simulink model "Controlled_simulink_model_optimal"  (R2017b)
settings: Solver=VariableStepAuto  StartTime=0  StopTime=5  FixedStep=0.001  MaxStep=1e-3  MinStep=1e-4  RelTol=1e-5
values from neighbouring files (symbols this model uses):
  Accel_bias = 0    [Controlled_model.m]
  Ax = 0.0    (= 0)    [Controlled_model.m]
  Ay = 0.0    (= 0)    [Controlled_model.m]
  b = 1.144e-08    [Controlled_model.m]
  d = 9.94e-10    [Controlled_model.m]
  g = 9.81    [Controlled_model.m]
  Gyro_bias = 0    [Controlled_model.m]
  Ixx = 7.5*10^(-3)    (= 0.0075)    [Controlled_model.m]
  Iyy = 7.5*10^(-3)    (= 0.0075)    [Controlled_model.m]
  Izz = 1.3*10^(-2)    (= 0.013)    [Controlled_model.m]
  Jr = 6.5*10^(-7)    (= 6.5e-07)    [Controlled_model.m]
  Kd = x(3)    [Controlled_model.m]    (also in OptPID.m)
  Ki = x(2)    [Controlled_model.m]    (also in OptPID.m)
  Kp = x(1)    [Controlled_model.m]    (also in OptPID.m)
  l = 0.23    [Controlled_model.m]
  m = weight/g    (= 0.0289500509684)    [Controlled_model.m]
libraries: simulink x1
settings Model: Creator=Nicky  LastModifiedBy=Nicky
settings SolverCC: MaxConsecutiveZCs=500  ZeroCrossAlgorithm=Adaptive  AlgebraicLoopSolver=LineSearch  AutoInsertRateTranBlk=on
settings DebuggingCC: MaxConsecutiveZCsMsg=none
settings CodeAppCC: StateflowObjectComments=on
settings SimscapeCC: SimscapeNormalizeSystem=off

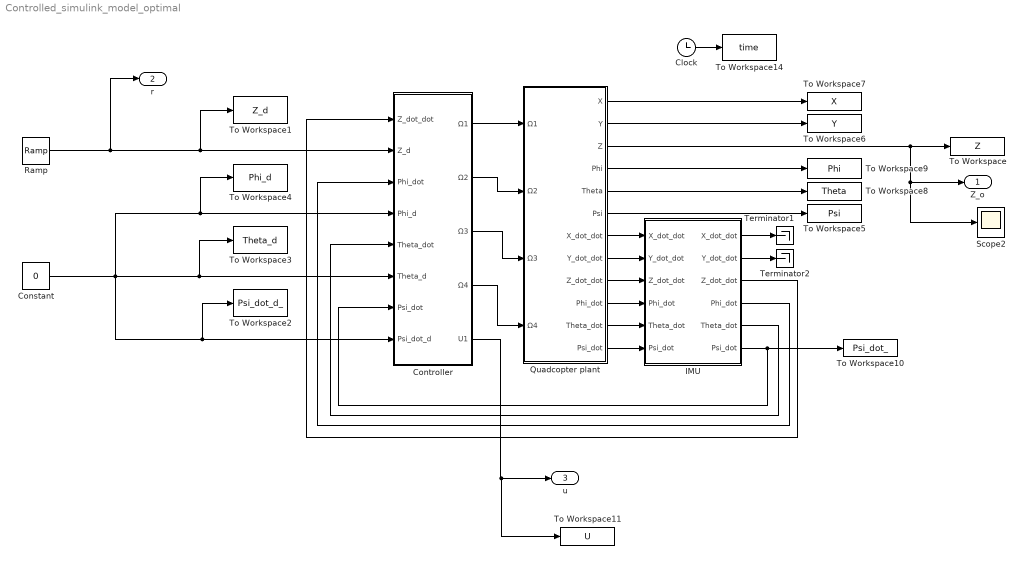
== system Controlled_simulink_model_optimal ==
  Clock : Clock
  Constant : Constant  Value=0
  Controller : Subsystem
  IMU : Subsystem
  Quadcopter plant : Subsystem
  Ramp : simulink/Sources/Ramp  slope=0  start=0  X0=-1
  Scope2 : Scope
  Terminator1 : Terminator
  Terminator2 : Terminator
  To Workspace : ToWorkspace  VariableName=Z  SampleTime=0.001
      settings: Save2DSignal=2-D array (concatenate along first dimension)
  To Workspace1 : ToWorkspace  VariableName=Z_d  SampleTime=0.001
      settings: Save2DSignal=2-D array (concatenate along first dimension)
  To Workspace10 : ToWorkspace  VariableName=Psi_dot_  SampleTime=0.001
      settings: Save2DSignal=2-D array (concatenate along first dimension)
  To Workspace11 : ToWorkspace  VariableName=U  SampleTime=0.001
      settings: Save2DSignal=2-D array (concatenate along first dimension)
  To Workspace14 : ToWorkspace  VariableName=time  SampleTime=0.001
      settings: Save2DSignal=2-D array (concatenate along first dimension)
  To Workspace2 : ToWorkspace  VariableName=Psi_dot_d_  SampleTime=0.001
      settings: Save2DSignal=2-D array (concatenate along first dimension)
  To Workspace3 : ToWorkspace  VariableName=Theta_d  SampleTime=0.001
      settings: Save2DSignal=2-D array (concatenate along first dimension)
  To Workspace4 : ToWorkspace  VariableName=Phi_d  SampleTime=0.001
      settings: Save2DSignal=2-D array (concatenate along first dimension)
  To Workspace5 : ToWorkspace  VariableName=Psi  SampleTime=0.001
      settings: Save2DSignal=2-D array (concatenate along first dimension)
  To Workspace6 : ToWorkspace  VariableName=Y  SampleTime=0.001
      settings: Save2DSignal=2-D array (concatenate along first dimension)
  To Workspace7 : ToWorkspace  VariableName=X  SampleTime=0.001
      settings: Save2DSignal=2-D array (concatenate along first dimension)
  To Workspace8 : ToWorkspace  VariableName=Theta  SampleTime=0.001
      settings: Save2DSignal=2-D array (concatenate along first dimension)
  To Workspace9 : ToWorkspace  VariableName=Phi  SampleTime=0.001
      settings: Save2DSignal=2-D array (concatenate along first dimension)
  Z_o : Outport
  r : Outport  Port=2
  "u " : Outport  Port=3
  wires:
  Clock/1 -> To Workspace14/1
  Controller/1(Ω1) -> Quadcopter plant/1(Ω1)
  Controller/2(Ω2) -> Quadcopter plant/2(Ω2)
  Controller/3(Ω3) -> Quadcopter plant/3(Ω3)
  Controller/4(Ω4) -> Quadcopter plant/4(Ω4)
  IMU/6("Psi_dot ") -> Controller/7(Psi_dot), To Workspace10/1
  IMU/5("Theta_dot ") -> Controller/5(Theta_dot)
  IMU/3("Z_dot_dot ") -> Controller/1(Z_dot_dot)
  Quadcopter plant/1(X) -> To Workspace7/1
  Quadcopter plant/2(Y) -> To Workspace6/1
  Quadcopter plant/7(X_dot_dot) -> IMU/1(X_dot_dot)
  Quadcopter plant/8("Y_dot_dot ") -> IMU/2(Y_dot_dot)
  Quadcopter plant/9(Z_dot_dot) -> IMU/3(Z_dot_dot)
  Quadcopter plant/11(Theta_dot) -> IMU/5(Theta_dot)
  Quadcopter plant/10(Phi_dot) -> IMU/4(Phi_dot)
  Quadcopter plant/12(Psi_dot) -> IMU/6(Psi_dot)
  Quadcopter plant/5(Theta) -> To Workspace8/1
  Quadcopter plant/6(Psi) -> To Workspace5/1
  IMU/1("X_dot_dot ") -> Terminator1/1
  IMU/2("Y_dot_dot ") -> Terminator2/1
  Constant/1 -> To Workspace4/1, Controller/4(Phi_d), To Workspace2/1, Controller/8(Psi_dot_d), To Workspace3/1, Controller/6(Theta_d)
  IMU/4("Phi_dot ") -> Controller/3(Phi_dot)
  Quadcopter plant/4(Phi) -> To Workspace9/1
  Ramp/1 -> r/1, To Workspace1/1, Controller/2(Z_d)
  Controller/5(U1) -> To Workspace11/1, "u "/1
  Quadcopter plant/3(Z) -> Z_o/1, Scope2/1, To Workspace/1

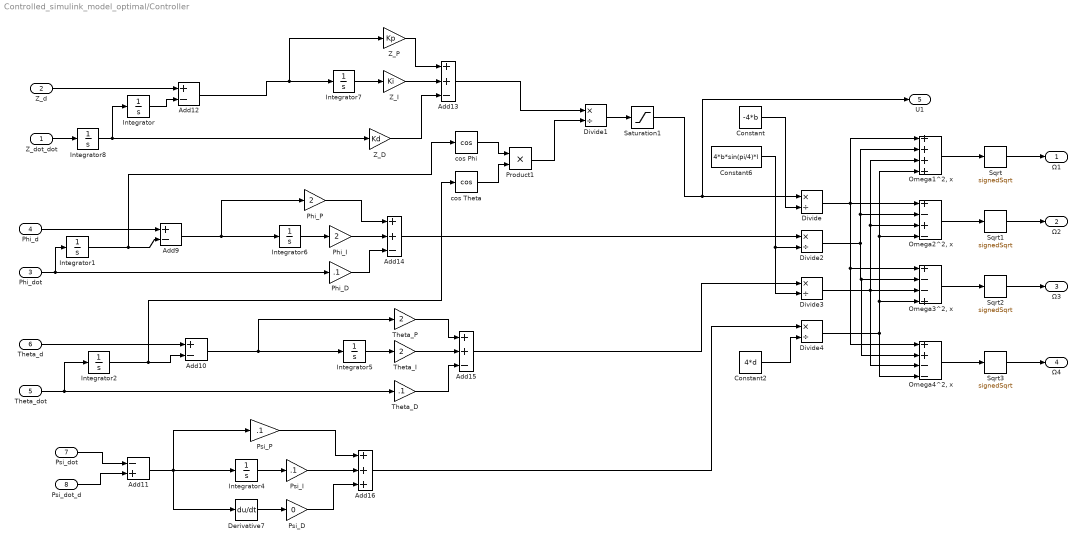
== system Controlled_simulink_model_optimal/Controller ==
  Z_dot_dot : Inport
  Z_d : Inport  Port=2
  Phi_dot : Inport  Port=3
  Phi_d : Inport  Port=4
  Theta_dot : Inport  Port=5
  Theta_d : Inport  Port=6
  Psi_dot : Inport  Port=7
  Psi_dot_d : Inport  Port=8
  Add10 : Sum  Inputs=+-
  Add11 : Sum  Inputs=-+
  Add12 : Sum  Inputs=+-
  Add13 : Sum  Inputs=++-
  Add14 : Sum  Inputs=++-
  Add15 : Sum  Inputs=++-
  Add16 : Sum  Inputs=+++
  Add9 : Sum  Inputs=+-
  Constant : Constant  Value=-4*b
  Constant2 : Constant  Value=4*d
  Constant6 : Constant  Value=4*b*sin(pi/4)*l
  Derivative7 : Derivative
  Divide{,1..4} (5 alike) : Product  Inputs=*/
  Integrator : Integrator  LimitOutput=on  UpperSaturationLimit=0
  Integrator1 : Integrator  WrapState=on
  Integrator2 : Integrator  WrapState=on
  Integrator{4..8} (5 alike) : Integrator
  "Omega1^2, x" : Sum  Inputs=++++
  "Omega2^2, x" : Sum  Inputs=+-+-
  "Omega3^2, x" : Sum  Inputs=+--+
  "Omega4^2, x" : Sum  Inputs=++--
  Phi_D : Gain  Gain=.1
  Phi_I : Gain  Gain=2
  Phi_P : Gain  Gain=2
  Product1 : Product  RndMeth=Zero
  Psi_D : Gain  Gain=0
  Psi_I : Gain  Gain=.1
  Psi_P : Gain  Gain=.1
  Saturation1 : Saturate  UpperLimit=0  LowerLimit=-inf
  Sqrt{,1..3} (4 alike) : Sqrt  Operator=signedSqrt  SaturateOnIntegerOverflow=on
  Theta_D : Gain  Gain=.1
  Theta_I : Gain  Gain=2
  Theta_P : Gain  Gain=2
  Z_D : Gain  Gain=Kd
  "Z_I " : Gain  Gain=Ki
  Z_P : Gain  Gain=Kp
  cos Phi : Trigonometry  Operator=cos
  cos Theta : Trigonometry  Operator=cos
  Ω1 : Outport
  Ω2 : Outport  Port=2
  Ω3 : Outport  Port=3
  Ω4 : Outport  Port=4
  U1 : Outport  Port=5
  wires:
  Z_D/1 -> Add13/3
  Theta_I/1 -> Add15/2
  Add12/1 -> Z_P/1, Integrator7/1
  Z_dot_dot/1 -> Integrator8/1
  Add11/1 -> Derivative7/1, Integrator4/1, Psi_P/1
  "Z_I "/1 -> Add13/2
  Theta_P/1 -> Add15/1
  Integrator4/1 -> Psi_I/1
  Integrator7/1 -> "Z_I "/1
  Add9/1 -> Integrator6/1, Phi_P/1
  Derivative7/1 -> Psi_D/1
  Psi_D/1 -> Add16/3
  Psi_I/1 -> Add16/2
  Integrator6/1 -> Phi_I/1
  cos Theta/1 -> Product1/2
  Add13/1 -> Divide1/1
  Phi_dot/1 -> Phi_D/1, Integrator1/1
  Phi_D/1 -> Add14/3
  cos Phi/1 -> Product1/1
  Divide1/1 -> Saturation1/1
  Theta_D/1 -> Add15/3
  Integrator5/1 -> Theta_I/1
  Add10/1 -> Theta_P/1, Integrator5/1
  Product1/1 -> Divide1/2
  Phi_I/1 -> Add14/2
  Theta_dot/1 -> Integrator2/1, Theta_D/1
  Phi_P/1 -> Add14/1
  Psi_P/1 -> Add16/1
  Z_P/1 -> Add13/1
  Constant6/1 -> Divide3/2, Divide2/2
  Add14/1 -> Divide2/1
  Add15/1 -> Divide3/1
  Saturation1/1 -> U1/1, Divide/1
  Constant/1 -> Divide/2
  Constant2/1 -> Divide4/2
  Add16/1 -> Divide4/1
  Sqrt/1 -> Ω1/1
  Sqrt1/1 -> Ω2/1
  Sqrt2/1 -> Ω3/1
  Sqrt3/1 -> Ω4/1
  Divide4/1 -> "Omega3^2, x"/4, "Omega2^2, x"/4, "Omega1^2, x"/4, "Omega4^2, x"/4
  Divide2/1 -> "Omega4^2, x"/2, "Omega3^2, x"/2, "Omega2^2, x"/2, "Omega1^2, x"/2
  Divide3/1 -> "Omega4^2, x"/3, "Omega3^2, x"/3, "Omega2^2, x"/3, "Omega1^2, x"/3
  Divide/1 -> "Omega4^2, x"/1, "Omega3^2, x"/1, "Omega2^2, x"/1, "Omega1^2, x"/1
  "Omega1^2, x"/1 -> Sqrt/1
  "Omega2^2, x"/1 -> Sqrt1/1
  "Omega3^2, x"/1 -> Sqrt2/1
  "Omega4^2, x"/1 -> Sqrt3/1
  Z_d/1 -> Add12/1
  Phi_d/1 -> Add9/1
  Integrator1/1 -> cos Phi/1, Add9/2
  Integrator2/1 -> cos Theta/1, Add10/2
  Theta_d/1 -> Add10/1
  Psi_dot/1 -> Add11/1
  Psi_dot_d/1 -> Add11/2
  Integrator/1 -> Add12/2
  Integrator8/1 -> Z_D/1, Integrator/1

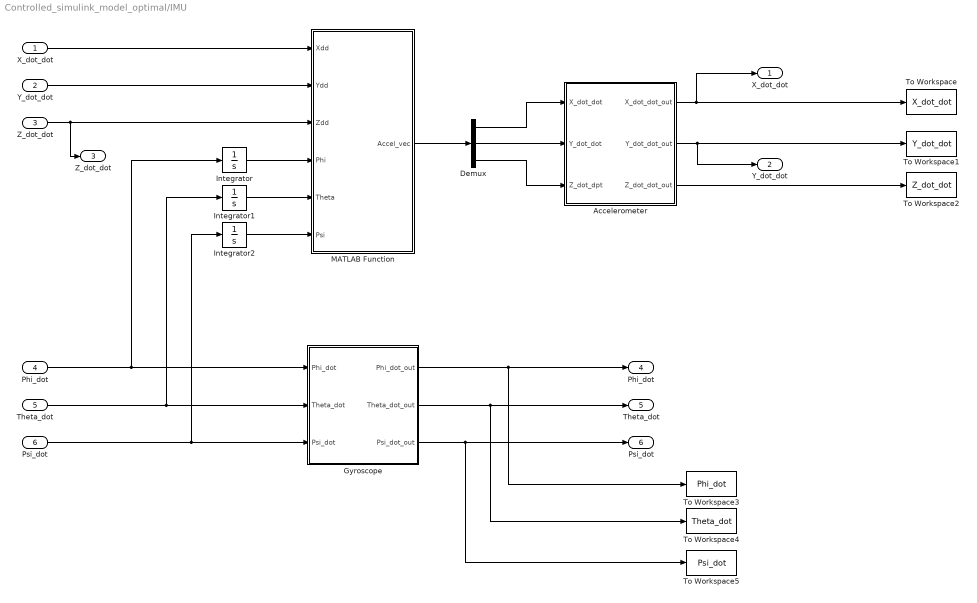
== system Controlled_simulink_model_optimal/IMU ==
  X_dot_dot : Inport
  Y_dot_dot : Inport  Port=2
  Z_dot_dot : Inport  Port=3
  Phi_dot : Inport  Port=4
  Theta_dot : Inport  Port=5
  Psi_dot : Inport  Port=6
  Accelerometer : Subsystem
  Demux : Demux  Outputs=3
  Gyroscope : Subsystem
  Integrator : Integrator  WrapState=on
  Integrator1 : Integrator  WrapState=on
  Integrator2 : Integrator
  MATLAB Function : MATLAB Function  TreatAsAtomicUnit=on
  To Workspace : ToWorkspace  VariableName=X_dot_dot  SampleTime=0.001
      settings: Save2DSignal=2-D array (concatenate along first dimension)
  To Workspace1 : ToWorkspace  VariableName=Y_dot_dot  SampleTime=0.001
      settings: Save2DSignal=2-D array (concatenate along first dimension)
  To Workspace2 : ToWorkspace  VariableName=Z_dot_dot  SampleTime=0.001
      settings: Save2DSignal=2-D array (concatenate along first dimension)
  To Workspace3 : ToWorkspace  VariableName=Phi_dot  SampleTime=0.001
      settings: Save2DSignal=2-D array (concatenate along first dimension)
  To Workspace4 : ToWorkspace  VariableName=Theta_dot  SampleTime=0.001
      settings: Save2DSignal=2-D array (concatenate along first dimension)
  To Workspace5 : ToWorkspace  VariableName=Psi_dot  SampleTime=0.001
      settings: Save2DSignal=2-D array (concatenate along first dimension)
  "X_dot_dot " : Outport
  "Y_dot_dot " : Outport  Port=2
  "Z_dot_dot " : Outport  Port=3
  "Phi_dot " : Outport  Port=4
  "Theta_dot " : Outport  Port=5
  "Psi_dot " : Outport  Port=6
  wires:
  Phi_dot/1 -> Integrator/1, Gyroscope/1(Phi_dot)
  Theta_dot/1 -> Integrator1/1, Gyroscope/2(Theta_dot)
  Psi_dot/1 -> Integrator2/1, Gyroscope/3(Psi_dot)
  Gyroscope/2(Theta_dot_out) -> "Theta_dot "/1, To Workspace4/1
  Gyroscope/1(Phi_dot_out) -> "Phi_dot "/1, To Workspace3/1
  Accelerometer/1(X_dot_dot_out) -> To Workspace/1, "X_dot_dot "/1
  Accelerometer/2(Y_dot_dot_out) -> To Workspace1/1, "Y_dot_dot "/1
  Accelerometer/3(Z_dot_dot_out) -> To Workspace2/1
  Gyroscope/3(Psi_dot_out) -> "Psi_dot "/1, To Workspace5/1
  X_dot_dot/1 -> MATLAB Function/1(Xdd)
  Y_dot_dot/1 -> MATLAB Function/2(Ydd)
  Z_dot_dot/1 -> "Z_dot_dot "/1, MATLAB Function/3(Zdd)
  Integrator/1 -> MATLAB Function/4(Phi)
  Integrator2/1 -> MATLAB Function/6(Psi)
  Integrator1/1 -> MATLAB Function/5(Theta)
  MATLAB Function/1(Accel_vec) -> Demux/1
  Demux/2 -> Accelerometer/2("Y_dot_dot ")
  Demux/1 -> Accelerometer/1(X_dot_dot)
  Demux/3 -> Accelerometer/3("Z_dot_dpt ")

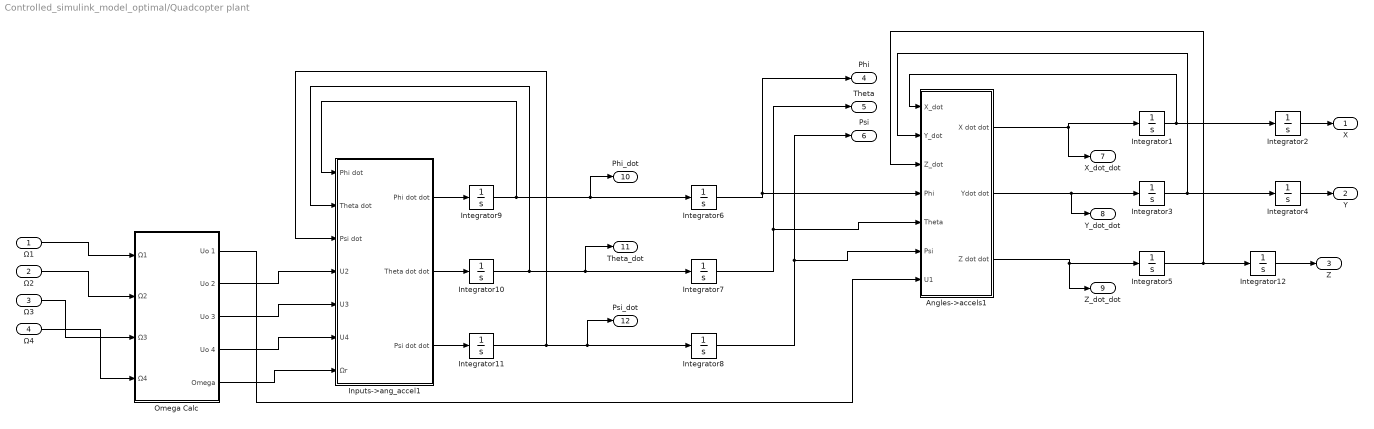
== system Controlled_simulink_model_optimal/Quadcopter plant ==
  Ω1 : Inport
  Ω2 : Inport  Port=2
  Ω3 : Inport  Port=3
  Ω4 : Inport  Port=4
  Angles->accels1 : Subsystem
  Inputs->ang_accel1 : Subsystem
  Integrator{1..5,8..9} (7 alike) : Integrator
  Integrator10 : Integrator  IgnoreLimit=on
  Integrator11 : Integrator  UpperSaturationLimit=10000  LowerSaturationLimit=-10000
  Integrator12 : Integrator  LimitOutput=on  UpperSaturationLimit=0
  Integrator6 : Integrator  WrapState=on
  Integrator7 : Integrator  WrapState=on
  Omega Calc : Subsystem
  X : Outport
  Y : Outport  Port=2
  Z : Outport  Port=3
  Phi : Outport  Port=4
  Theta : Outport  Port=5
  Psi : Outport  Port=6
  X_dot_dot : Outport  Port=7
  "Y_dot_dot " : Outport  Port=8
  Z_dot_dot : Outport  Port=9
  Phi_dot : Outport  Port=10
  Theta_dot : Outport  Port=11
  Psi_dot : Outport  Port=12
  wires:
  Integrator7/1 -> Angles->accels1/5(Theta), Theta/1
  Integrator6/1 -> Angles->accels1/4(Phi), Phi/1
  Inputs->ang_accel1/2(Theta dot dot) -> Integrator10/1
  Inputs->ang_accel1/1(Phi dot dot) -> Integrator9/1
  Inputs->ang_accel1/3(Psi dot dot) -> Integrator11/1
  Omega Calc/5(Omega) -> Inputs->ang_accel1/7(Ωr)
  Omega Calc/4(Uo 4) -> Inputs->ang_accel1/6(U4)
  Omega Calc/3(Uo 3) -> Inputs->ang_accel1/5(U3)
  Omega Calc/2(Uo 2) -> Inputs->ang_accel1/4(U2)
  Omega Calc/1(Uo 1) -> Angles->accels1/7(U1)
  Ω1/1 -> Omega Calc/1(Ω1)
  Ω2/1 -> Omega Calc/2(Ω2)
  Ω3/1 -> Omega Calc/3(Ω3)
  Ω4/1 -> Omega Calc/4(Ω4)
  Integrator9/1 -> Inputs->ang_accel1/1(Phi dot), Phi_dot/1, Integrator6/1
  Integrator11/1 -> Inputs->ang_accel1/3(Psi dot), Integrator8/1, Psi_dot/1
  Integrator10/1 -> Inputs->ang_accel1/2(Theta dot), Integrator7/1, Theta_dot/1
  Angles->accels1/1(X dot dot) -> X_dot_dot/1, Integrator1/1
  Integrator1/1 -> Angles->accels1/1(X_dot), Integrator2/1
  Integrator2/1 -> X/1
  Integrator3/1 -> Angles->accels1/2(Y_dot), Integrator4/1
  Angles->accels1/2(Ydot dot) -> "Y_dot_dot "/1, Integrator3/1
  Integrator4/1 -> Y/1
  Integrator5/1 -> Angles->accels1/3(Z_dot), Integrator12/1
  Angles->accels1/3(Z dot dot) -> Integrator5/1, Z_dot_dot/1
  Integrator12/1 -> Z/1
  Integrator8/1 -> Angles->accels1/6(Psi), Psi/1

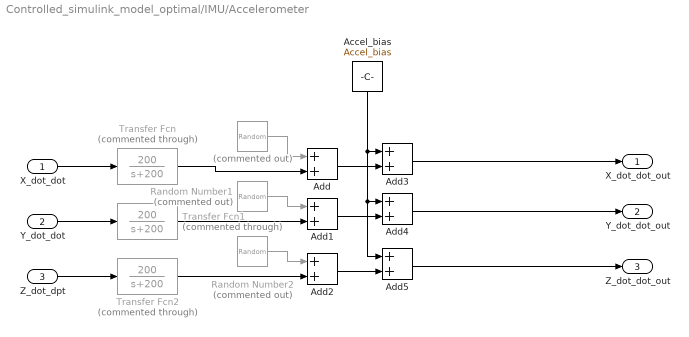
== system Controlled_simulink_model_optimal/IMU/Accelerometer ==
  X_dot_dot : Inport
  "Y_dot_dot " : Inport  Port=2
  "Z_dot_dpt " : Inport  Port=3
  " " : RandomNumber  Commented=on  Variance=0.0001  Seed=1  SampleTime=0.001
  Accel_bias : Constant  Value=Accel_bias
  Add{,1..5} (6 alike) : Sum
  Random Number1 : RandomNumber  Commented=on  Variance=0.0001  Seed=2  SampleTime=0.001
  Random Number2 : RandomNumber  Commented=on  Mean=0.000  Variance=0.0001  Seed=3  SampleTime=0.001
  Transfer Fcn : TransferFcn  Commented=through  Numerator=[200]  Denominator=[1 200]
  Transfer Fcn1 : TransferFcn  Commented=through  Numerator=[200]  Denominator=[1 200]
  Transfer Fcn2 : TransferFcn  Commented=through  Numerator=[200]  Denominator=[1 200]
  X_dot_dot_out : Outport
  Y_dot_dot_out : Outport  Port=2
  Z_dot_dot_out : Outport  Port=3
  wires:
  X_dot_dot/1 -> Transfer Fcn/1
  "Y_dot_dot "/1 -> Transfer Fcn1/1
  Accel_bias/1 -> Add5/1, Add4/1, Add3/1
  Add/1 -> Add3/2
  Add2/1 -> Add5/2
  Add1/1 -> Add4/2
  " "/1 -> Add/1
  Random Number1/1 -> Add1/1
  Random Number2/1 -> Add2/1
  "Z_dot_dpt "/1 -> Transfer Fcn2/1
  Add3/1 -> X_dot_dot_out/1
  Add4/1 -> Y_dot_dot_out/1
  Add5/1 -> Z_dot_dot_out/1
  Transfer Fcn/1 -> Add/2
  Transfer Fcn1/1 -> Add1/2
  Transfer Fcn2/1 -> Add2/2

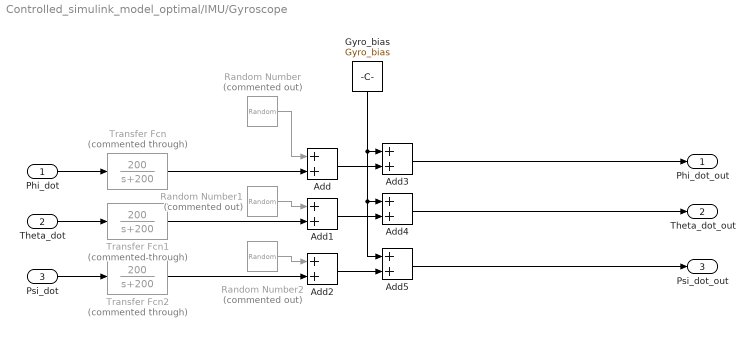
== system Controlled_simulink_model_optimal/IMU/Gyroscope ==
  Phi_dot : Inport
  Theta_dot : Inport  Port=2
  Psi_dot : Inport  Port=3
  Add{,1..5} (6 alike) : Sum
  Gyro_bias : Constant  Value=Gyro_bias
  Random Number : RandomNumber  Commented=on  Variance=0.0001  Seed=4  SampleTime=0.001
  Random Number1 : RandomNumber  Commented=on  Variance=0.0001  Seed=5  SampleTime=0.001
  Random Number2 : RandomNumber  Commented=on  Variance=0.0001  Seed=6  SampleTime=0.001
  Transfer Fcn : TransferFcn  Commented=through  Numerator=[200]  Denominator=[1 200]
  Transfer Fcn1 : TransferFcn  Commented=through  Numerator=[200]  Denominator=[1 200]
  Transfer Fcn2 : TransferFcn  Commented=through  Numerator=[200]  Denominator=[1 200]
  Phi_dot_out : Outport
  Theta_dot_out : Outport  Port=2
  Psi_dot_out : Outport  Port=3
  wires:
  Phi_dot/1 -> Transfer Fcn/1
  Theta_dot/1 -> Transfer Fcn1/1
  Psi_dot/1 -> Transfer Fcn2/1
  Add/1 -> Add3/2
  Add1/1 -> Add4/2
  Add2/1 -> Add5/2
  Gyro_bias/1 -> Add5/1, Add4/1, Add3/1
  Random Number/1 -> Add/1
  Random Number1/1 -> Add1/1
  Random Number2/1 -> Add2/1
  Add3/1 -> Phi_dot_out/1
  Add4/1 -> Theta_dot_out/1
  Add5/1 -> Psi_dot_out/1
  Transfer Fcn2/1 -> Add2/2
  Transfer Fcn1/1 -> Add1/2
  Transfer Fcn/1 -> Add/2

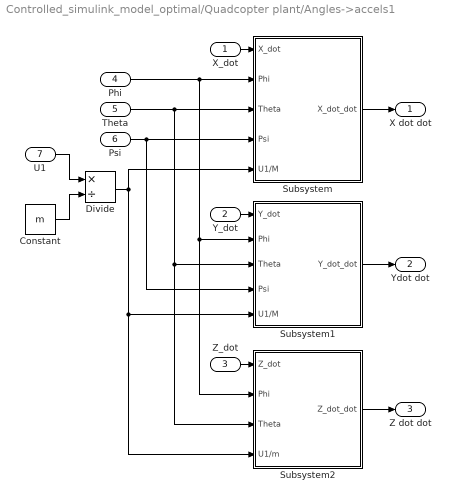
== system Controlled_simulink_model_optimal/Quadcopter plant/Angles->accels1 ==
  X_dot : Inport
  Y_dot : Inport  Port=2
  Z_dot : Inport  Port=3
  Phi : Inport  Port=4
  Theta : Inport  Port=5
  Psi : Inport  Port=6
  U1 : Inport  Port=7
  Constant : Constant  Value=m
  Divide : Product  Inputs=*/
  Subsystem : Subsystem
  Subsystem1 : Subsystem
  Subsystem2 : Subsystem
  X dot dot : Outport
  Ydot dot : Outport  Port=2
  Z dot dot : Outport  Port=3
  wires:
  Phi/1 -> Subsystem2/2(Phi), Subsystem1/2(Phi), Subsystem/2(Phi)
  U1/1 -> Divide/1
  Constant/1 -> Divide/2
  Divide/1 -> Subsystem/5(U1/M), Subsystem2/4(U1/m), Subsystem1/5(U1/M)
  Subsystem/1(X_dot_dot) -> X dot dot/1
  Subsystem1/1(Y_dot_dot) -> Ydot dot/1
  Subsystem2/1(Z_dot_dot) -> Z dot dot/1
  Theta/1 -> Subsystem2/3(Theta), Subsystem1/3(Theta), Subsystem/3(Theta)
  Psi/1 -> Subsystem1/4(Psi), Subsystem/4(Psi)
  X_dot/1 -> Subsystem/1(X_dot)
  Y_dot/1 -> Subsystem1/1(Y_dot)
  Z_dot/1 -> Subsystem2/1(Z_dot)

== system Controlled_simulink_model_optimal/Quadcopter plant/Inputs->ang_accel1 ==
  Phi dot : Inport
  Theta dot : Inport  Port=2
  Psi dot : Inport  Port=3
  U2 : Inport  Port=4
  U3 : Inport  Port=5
  U4 : Inport  Port=6
  Ωr : Inport  Port=7
  Subsystem : Subsystem
  Subsystem1 : Subsystem
  Subsystem2 : Subsystem
  Phi dot dot : Outport
  Theta dot dot : Outport  Port=2
  Psi dot dot : Outport  Port=3
  wires:
  U3/1 -> Subsystem2/3(U3)
  U4/1 -> Subsystem1/3(U4)
  Subsystem/1(Phi_dot_dot) -> Phi dot dot/1
  U2/1 -> Subsystem/1(U2)
  Ωr/1 -> Subsystem/4(Ωr), Subsystem2/1(Ωr)
  Psi dot/1 -> Subsystem2/2(Psi_dot), Subsystem/3(Psi_dot)
  Subsystem2/1(Theta_dot_dot) -> Theta dot dot/1
  Subsystem1/1(Psi_dot_dot) -> Psi dot dot/1
  Theta dot/1 -> Subsystem/2(Theta_dot), Subsystem1/2(Theta_dot)
  Phi dot/1 -> Subsystem2/4(Phi_dot), Subsystem1/1(Phi_dot)

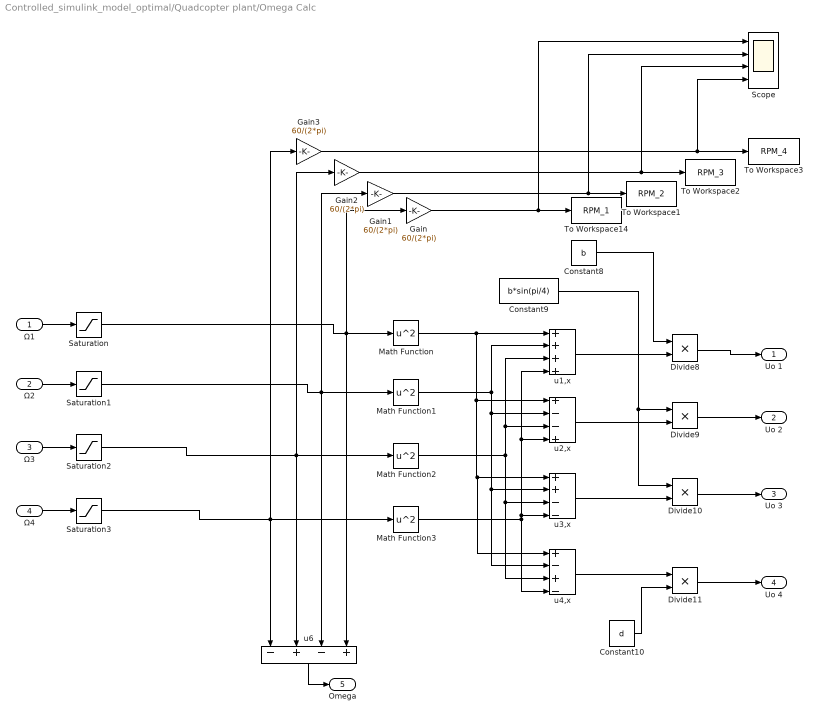
== system Controlled_simulink_model_optimal/Quadcopter plant/Omega Calc ==
  Ω1 : Inport
  Ω2 : Inport  Port=2
  Ω3 : Inport  Port=3
  Ω4 : Inport  Port=4
  Constant10 : Constant  Value=d
  Constant8 : Constant  Value=b
  Constant9 : Constant  Value=b*sin(pi/4)
  Divide{8..11} (4 alike) : Product  Inputs=**
  Gain{,1..3} (4 alike) : Gain  Gain=60/(2*pi)
  Math Function{,1..3} (4 alike) : Math  Operator=square  SaturateOnIntegerOverflow=on
  Saturation{,1..3} (4 alike) : Saturate  UpperLimit=inf  LowerLimit=0
  Scope : Scope  NumInputPorts=4
  To Workspace1 : ToWorkspace  VariableName=RPM_2  SampleTime=0.001
      settings: Save2DSignal=2-D array (concatenate along first dimension)
  To Workspace14 : ToWorkspace  VariableName=RPM_1  SampleTime=0.001
      settings: Save2DSignal=2-D array (concatenate along first dimension)
  To Workspace2 : ToWorkspace  VariableName=RPM_3  SampleTime=0.001
      settings: Save2DSignal=2-D array (concatenate along first dimension)
  To Workspace3 : ToWorkspace  VariableName=RPM_4  SampleTime=0.001
      settings: Save2DSignal=2-D array (concatenate along first dimension)
  u1,x : Sum  Inputs=++++
  u2,x : Sum  Inputs=+--+
  u3,x : Sum  Inputs=++--
  u4,x : Sum  Inputs=+-+-
  u6 : Sum  Inputs=-+-+
  Uo 1 : Outport
  Uo 2 : Outport  Port=2
  Uo 3 : Outport  Port=3
  Uo 4 : Outport  Port=4
  Omega : Outport  Port=5
  wires:
  Constant10/1 -> Divide11/2
  u4,x/1 -> Divide11/1
  u3,x/1 -> Divide10/2
  u2,x/1 -> Divide9/2
  Constant9/1 -> Divide10/1, Divide9/1
  u1,x/1 -> Divide8/2
  Constant8/1 -> Divide8/1
  u6/1 -> Omega/1
  Divide8/1 -> Uo 1/1
  Divide9/1 -> Uo 2/1
  Divide10/1 -> Uo 3/1
  Divide11/1 -> Uo 4/1
  Saturation/1 -> Gain/1, u6/4, Math Function/1
  Saturation1/1 -> Gain1/1, u6/3, Math Function1/1
  Saturation2/1 -> Math Function2/1, Gain2/1, u6/2
  Saturation3/1 -> Math Function3/1, Gain3/1, u6/1
  Ω1/1 -> Saturation/1
  Ω2/1 -> Saturation1/1
  Ω3/1 -> Saturation2/1
  Ω4/1 -> Saturation3/1
  Math Function/1 -> u4,x/1, u3,x/1, u2,x/1, u1,x/1
  Math Function1/1 -> u4,x/2, u3,x/2, u2,x/2, u1,x/2
  Math Function2/1 -> u4,x/3, u3,x/3, u1,x/3, u2,x/3
  Math Function3/1 -> u4,x/4, u1,x/4, u2,x/4, u3,x/4
  Gain/1 -> Scope/1, To Workspace14/1
  Gain1/1 -> Scope/2, To Workspace1/1
  Gain2/1 -> Scope/3, To Workspace2/1
  Gain3/1 -> Scope/4, To Workspace3/1

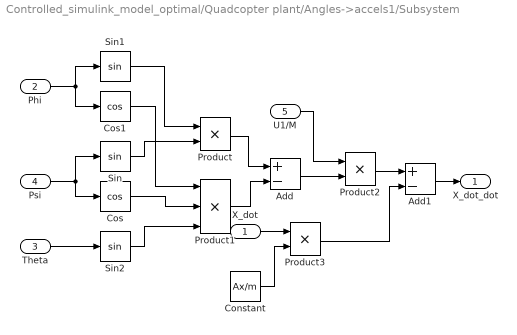
== system Controlled_simulink_model_optimal/Quadcopter plant/Angles->accels1/Subsystem ==
  X_dot : Inport
  Phi : Inport  Port=2
  Theta : Inport  Port=3
  Psi : Inport  Port=4
  U1/M : Inport  Port=5
  Add : Sum  Inputs=+-
  Add1 : Sum  Inputs=+-
  Constant : Constant  Value=Ax/m
  Cos : Trigonometry  Operator=cos
  Cos1 : Trigonometry  Operator=cos
  Product : Product
  Product1 : Product  Inputs=3
  Product2 : Product
  Product3 : Product
  Sin : Trigonometry
  Sin1 : Trigonometry
  Sin2 : Trigonometry
  X_dot_dot : Outport
  wires:
  Product1/1 -> Add/2
  Product/1 -> Add/1
  U1/M/1 -> Product2/1
  Add/1 -> Product2/2
  Psi/1 -> Cos/1, Sin/1
  Phi/1 -> Cos1/1, Sin1/1
  Theta/1 -> Sin2/1
  Cos1/1 -> Product1/1
  Cos/1 -> Product1/2
  Sin2/1 -> Product1/3
  Sin1/1 -> Product/1
  Sin/1 -> Product/2
  Product2/1 -> Add1/1
  Add1/1 -> X_dot_dot/1
  X_dot/1 -> Product3/1
  Constant/1 -> Product3/2
  Product3/1 -> Add1/2

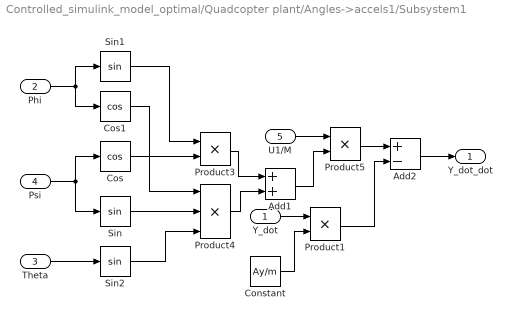
== system Controlled_simulink_model_optimal/Quadcopter plant/Angles->accels1/Subsystem1 ==
  Y_dot : Inport
  Phi : Inport  Port=2
  Theta : Inport  Port=3
  Psi : Inport  Port=4
  U1/M : Inport  Port=5
  Add1 : Sum
  Add2 : Sum  Inputs=+-
  Constant : Constant  Value=Ay/m
  Cos : Trigonometry  Operator=cos
  Cos1 : Trigonometry  Operator=cos
  Product1 : Product
  Product3 : Product
  Product4 : Product  Inputs=3
  Product5 : Product
  Sin : Trigonometry
  Sin1 : Trigonometry
  Sin2 : Trigonometry
  Y_dot_dot : Outport
  wires:
  Psi/1 -> Sin/1, Cos/1
  Phi/1 -> Cos1/1, Sin1/1
  Theta/1 -> Sin2/1
  Add1/1 -> Product5/2
  Product4/1 -> Add1/2
  U1/M/1 -> Product5/1
  Product3/1 -> Add1/1
  Cos1/1 -> Product4/1
  Sin/1 -> Product4/2
  Sin2/1 -> Product4/3
  Sin1/1 -> Product3/1
  Cos/1 -> Product3/2
  Y_dot/1 -> Product1/1
  Constant/1 -> Product1/2
  Product1/1 -> Add2/2
  Product5/1 -> Add2/1
  Add2/1 -> Y_dot_dot/1

== system Controlled_simulink_model_optimal/Quadcopter plant/Angles->accels1/Subsystem2 ==
  Z_dot : Inport
  Phi : Inport  Port=2
  Theta : Inport  Port=3
  U1/m : Inport  Port=4
  Add1 : Sum  Inputs=+-
  Add2 : Sum  Inputs=+-
  Constant : Constant  Value=Ay/m
  Constant2 : Constant  Value=g
  Cos : Trigonometry  Operator=cos
  Cos1 : Trigonometry  Operator=cos
  Product1 : Product
  Product6 : Product  Inputs=3
  Z_dot_dot : Outport
  wires:
  Phi/1 -> Cos1/1
  Theta/1 -> Cos/1
  U1/m/1 -> Product6/3
  Constant2/1 -> Add2/1
  Cos/1 -> Product6/1
  Product6/1 -> Add2/2
  Cos1/1 -> Product6/2
  Product1/1 -> Add1/2
  Z_dot/1 -> Product1/1
  Constant/1 -> Product1/2
  Add2/1 -> Add1/1
  Add1/1 -> Z_dot_dot/1

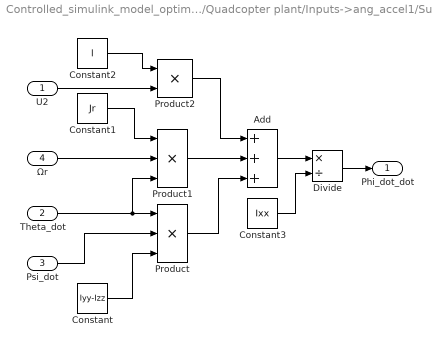
== system Controlled_simulink_model_optimal/Quadcopter plant/Inputs->ang_accel1/Subsystem ==
  U2 : Inport
  Theta_dot : Inport  Port=2
  Psi_dot : Inport  Port=3
  Ωr : Inport  Port=4
  Add : Sum  Inputs=+++
  Constant : Constant  Value=Iyy-Izz
  Constant1 : Constant  Value=Jr
  Constant2 : Constant  Value=l
  Constant3 : Constant  Value=Ixx
  Divide : Product  Inputs=*/
  Product : Product  Inputs=3
  Product1 : Product  Inputs=3
  Product2 : Product
  Phi_dot_dot : Outport
  wires:
  Psi_dot/1 -> Product/2
  Theta_dot/1 -> Product/1, Product1/3
  Constant/1 -> Product/3
  Ωr/1 -> Product1/2
  Constant1/1 -> Product1/1
  U2/1 -> Product2/2
  Constant2/1 -> Product2/1
  Product1/1 -> Add/2
  Product2/1 -> Add/1
  Product/1 -> Add/3
  Add/1 -> Divide/1
  Constant3/1 -> Divide/2
  Divide/1 -> Phi_dot_dot/1

== system Controlled_simulink_model_optimal/Quadcopter plant/Inputs->ang_accel1/Subsystem1 ==
  Phi_dot : Inport
  Theta_dot : Inport  Port=2
  U4 : Inport  Port=3
  Add2 : Sum
  Constant11 : Constant  Value=Izz
  Constant8 : Constant  Value=Ixx-Iyy
  Divide2 : Product  Inputs=*/
  Product6 : Product  Inputs=3
  Psi_dot_dot : Outport
  wires:
  Theta_dot/1 -> Product6/1
  Phi_dot/1 -> Product6/2
  Constant8/1 -> Product6/3
  Add2/1 -> Divide2/1
  Constant11/1 -> Divide2/2
  Divide2/1 -> Psi_dot_dot/1
  Product6/1 -> Add2/2
  U4/1 -> Add2/1

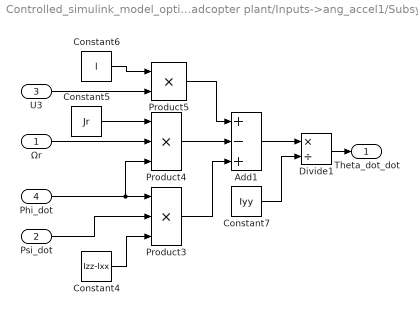
== system Controlled_simulink_model_optimal/Quadcopter plant/Inputs->ang_accel1/Subsystem2 ==
  Ωr : Inport
  Psi_dot : Inport  Port=2
  U3 : Inport  Port=3
  Phi_dot : Inport  Port=4
  Add1 : Sum  Inputs=+-+
  Constant4 : Constant  Value=Izz-Ixx
  Constant5 : Constant  Value=Jr
  Constant6 : Constant  Value=l
  Constant7 : Constant  Value=Iyy
  Divide1 : Product  Inputs=*/
  Product3 : Product  Inputs=3
  Product4 : Product  Inputs=3
  Product5 : Product
  Theta_dot_dot : Outport
  wires:
  Psi_dot/1 -> Product3/2
  Phi_dot/1 -> Product4/3, Product3/1
  Ωr/1 -> Product4/2
  Constant4/1 -> Product3/3
  Constant5/1 -> Product4/1
  U3/1 -> Product5/2
  Constant6/1 -> Product5/1
  Product4/1 -> Add1/2
  Product5/1 -> Add1/1
  Product3/1 -> Add1/3
  Add1/1 -> Divide1/1
  Constant7/1 -> Divide1/2
  Divide1/1 -> Theta_dot_dot/1

== matlab function Controlled_simulink_model_optimal/IMU/MATLAB Function ==
  data: Xdd input; Ydd input; Zdd input; Phi input; Accel_vec output; Theta input; Psi input
function Accel_vec = World2Body(Xdd,Ydd,Zdd,Phi,Theta,Psi)

Trans_mat=[(cos(Psi)*cos(Theta)), (-sin(Psi)*cos(Phi)+cos(Psi)*sin(Theta)*sin(Phi)), (sin(Psi)*sin(Phi)+cos(Psi)*sin(Theta)*cos(Phi));...
          (sin(Psi)*cos(Theta)), (cos(Psi)*cos(Phi)+sin(Theta)*sin(Psi)*sin(Phi)), (-cos(Psi)*sin(Phi)+sin(Theta)*sin(Psi)*cos(Phi));...
          (-sin(Theta)), (cos(Theta)*sin(Phi)), (cos(Theta)*cos(Phi))];
      
Accel_world=[Xdd;Ydd;Zdd];
Accel_vec=(Trans_mat^-1)*Accel_world;
